simulink model "simulink_observador"  (R2014b)
settings: Solver=ode45  StartTime=0.0  StopTime=25  MaxStep=0.001  RelTol=1e-3
values from neighbouring files (symbols this model uses):
  A = [0 -23.8095;0 0]    [Observador.m]    (also in P1.m; P1_pert.m; P1_pert_range.m; P1_pert_sin.m)
  B = [0;-23.8095]    [Observador.m]    (also in P1.m; P1_pert.m; P1_pert_range.m; P1_pert_sin.m)
  C = [1 0]    [Observador.m]    (also in P1.m; P1_pert.m = eye(2); P1_pert_range.m = eye(2); P1_pert_sin.m = eye(2))
  D = [0;0]    [Observador.m]    (also in P1.m; P1_pert.m; P1_pert_range.m; P1_pert_sin.m)
  gam = [0.708615362812 -1.190475]    [matlab.mat]
  K_dis = acker(phi,gam,P_dis)    [Observador.m]    (also in P1.m; P1_pert.m; P1_pert_range.m; P1_pert_sin.m)
  L = K_obs_dis'    [Observador.m]    (also in P1.m; fourier_plot.m = length(y); matlab.mat = [1.34458017196 -0.598466673493])
  phi = [1  -1.190475; 0  1]    [matlab.mat]
settings Model: Creator=student  LastModifiedBy=lluis
settings DataIOCC: SignalLoggingSaveFormat=ModelDataLogs
settings OptimizationCC: ExpressionDepthLimit=2147483647
settings DebuggingCC: UnderspecifiedInitializationDetection=Classic  MergeDetectMultiDrivingBlocksExec=none  FcnCallInpInsideContextMsg=EnableAllAsWarning  StateNameClashWarn=warning
settings GRTTargetCC: CombineOutputUpdateFcns=off  GRTInterface=on

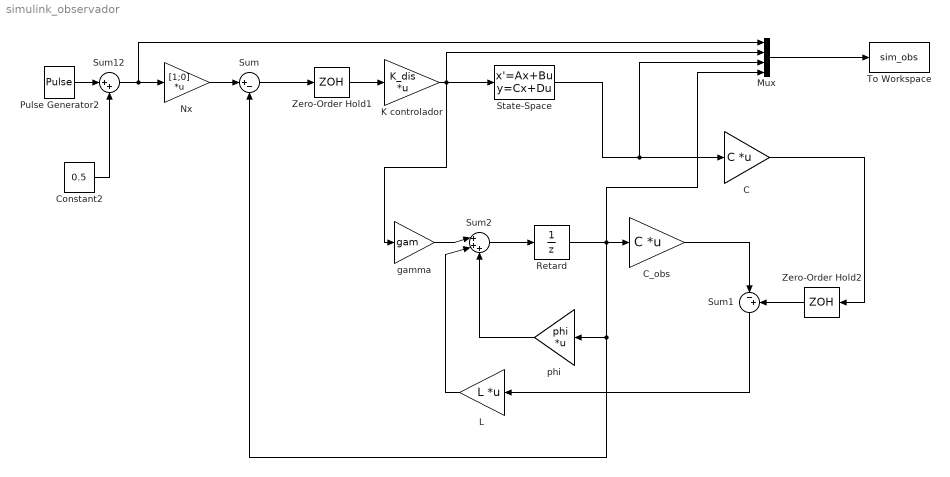
== system simulink_observador ==
  C : Gain  Gain=C  Multiplication=Matrix(K*u)
  C_obs : Gain  Gain=C  Multiplication=Matrix(K*u)
  Constant2 : Constant  Value=0.5
  K controlador : Gain  Gain=K_dis  Multiplication=Matrix(K*u)
  L : Gain  Gain=L  Multiplication=Matrix(K*u)
  Mux : Mux
  Nx : Gain  Gain=[1;0]  Multiplication=Matrix(K*u)
  Pulse Generator2 : DiscretePulseGenerator  PulseType=Time based  Amplitude=-2  Period=20  PulseWidth=50
  Retard : UnitDelay  SampleTime=-1
  State-Space : StateSpace  A=A  B=B  C=eye(2)  D=D  X0=[1;1]
  Sum : Sum  Inputs=|+-
  Sum1 : Sum  Inputs=|-+
  Sum12 : Sum  Inputs=|++
  Sum2 : Sum  Inputs=|+++
  To Workspace : ToWorkspace  VariableName=sim_obs  SaveFormat=Timeseries  SampleTime=-1
  Zero-Order Hold1 : ZeroOrderHold  SampleTime=5E-2
  Zero-Order Hold2 : ZeroOrderHold  SampleTime=5E-2
  gamma : Gain  Gain=gam
  phi : Gain  Gain=phi  Multiplication=Matrix(K*u)
  wires:
  State-Space/1 -> C/1, Mux/3
  Sum/1 -> Zero-Order Hold1/1
  Nx/1 -> Sum/1
  Zero-Order Hold1/1 -> K controlador/1
  Sum1/1 -> L/1
  gamma/1 -> Sum2/1
  L/1 -> Sum2/2
  Retard/1 -> C_obs/1, phi/1, Sum/2, Mux/4
  Sum2/1 -> Retard/1
  phi/1 -> Sum2/3
  C/1 -> Zero-Order Hold2/1
  C_obs/1 -> Sum1/1
  Mux/1 -> To Workspace/1
  K controlador/1 -> gamma/1, Mux/2, State-Space/1
  Zero-Order Hold2/1 -> Sum1/2
  Sum12/1 -> Mux/1, Nx/1
  Pulse Generator2/1 -> Sum12/1
  Constant2/1 -> Sum12/2
